simulink model "test_correlator"  (R2014b)
settings: Solver=ode45  StartTime=0.0  StopTime=3  RelTol=1e-3
libraries: siglabs_lib x1, simulink x1
settings Model: NumberOfSteps=1000  Creator=Ben  LastModifiedBy=Ben

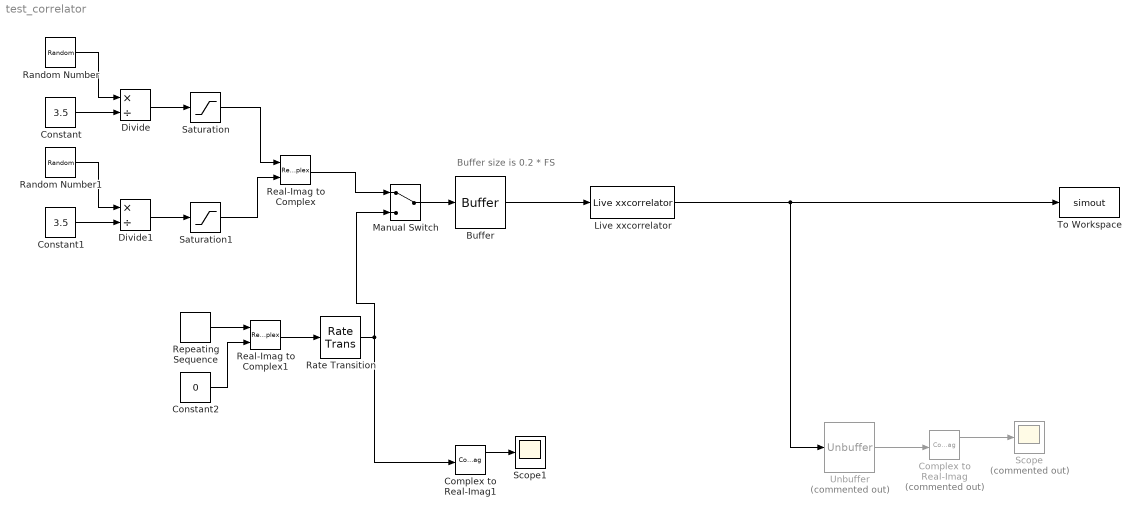
== system test_correlator ==
  note: Buffer size is 0.2 * FS
  Buffer : Buffer  N=25000  ic=11  TreatMby1Signals=One channel
  Complex to Real-Imag : ComplexToRealImag  Commented=on
  Complex to Real-Imag1 : ComplexToRealImag
  Constant : Constant  Value=3.5
  Constant1 : Constant  Value=3.5
  Constant2 : Constant  Value=0
  Divide : Product  Inputs=*/
  Divide1 : Product  Inputs=*/
  Live xxcorrelator : siglabs_lib/Live xxcorrelator  samps_per_second=125000
  Manual Switch : ManualSwitch
  Random Number : RandomNumber  SampleTime=1/125000
  Random Number1 : RandomNumber  SampleTime=1/125000
  Rate Transition : RateTransition  OutPortSampleTime=1/125000
  Real-Imag to Complex : RealImagToComplex
  Real-Imag to Complex1 : RealImagToComplex
  Repeating Sequence : simulink/Sources/Repeating Sequence  rep_seq_t=0.1*3:0.1*3:1*3  rep_seq_y=1:10
  Saturation : Saturate  UpperLimit=1  LowerLimit=-1
  Saturation1 : Saturate  UpperLimit=1  LowerLimit=-1
  Scope : Scope  Commented=on
      settings: YMin=-1  YMax=1
  Scope1 : Scope
      settings: YMin=0  YMax=10
  To Workspace : ToWorkspace  VariableName=simout  SampleTime=-1
      settings: Save2DSignal=2-D array (concatenate along first dimension)
  Unbuffer : Unbuffer  Commented=on  SampleBasedProcessing=Same as frame based
  wires:
  Constant/1 -> Divide/2
  Random Number/1 -> Divide/1
  Divide/1 -> Saturation/1
  Saturation/1 -> Real-Imag to Complex/1
  Constant1/1 -> Divide1/2
  Random Number1/1 -> Divide1/1
  Divide1/1 -> Saturation1/1
  Saturation1/1 -> Real-Imag to Complex/2
  Real-Imag to Complex/1 -> Manual Switch/1
  Buffer/1 -> Live xxcorrelator/1
  Live xxcorrelator/1 -> Unbuffer/1, To Workspace/1
  Manual Switch/1 -> Buffer/1
  Complex to Real-Imag/1 -> Scope/1
  Unbuffer/1 -> Complex to Real-Imag/1
  Constant2/1 -> Real-Imag to Complex1/2
  Repeating Sequence/1 -> Real-Imag to Complex1/1
  Real-Imag to Complex1/1 -> Rate Transition/1
  Rate Transition/1 -> Manual Switch/2, Complex to Real-Imag1/1
  Complex to Real-Imag1/1 -> Scope1/1
